simulink model "im1"  (R2018a)
settings: Solver=VariableStepAuto  StartTime=0.0  StopTime=10.0  RelTol=1e-3
values from neighbouring files (symbols this model uses):
  f = 0    [im.m]
  j = 0.011    [im.m]
  k = m/sigma/ls/lr    (= 95.8433439252)    [im.m]
  lambda = rs/sigma/ls+(1-sigma)/sigma/tr    (= 237.19971154)    [im.m]
  lr = 0.1164    [im.m]
  m = 0.1113    [im.m]
  p = 2    [im.m]
  tr = lr/rr    (= 0.111387559809)    [im.m]
settings Model: Creator=Yara  LastModifiedBy=Yara

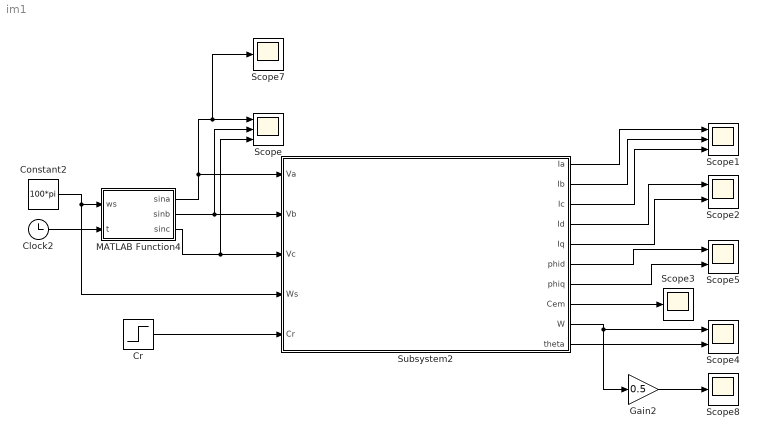
== system im1 ==
  Clock2 : Clock
  Constant2 : Constant  Value=100*pi
  Cr : Step  After=5  SampleTime=0
  Gain2 : Gain  Gain=0.5
  MATLAB Function4 : MATLAB Function  TreatAsAtomicUnit=on
  Scope : Scope  NumInputPorts=3
  Scope1 : Scope  NumInputPorts=3
  Scope2 : Scope  NumInputPorts=2
  Scope3 : Scope
  Scope4 : Scope  NumInputPorts=2
  Scope5 : Scope  NumInputPorts=2
  Scope7 : Scope
  Scope8 : Scope
  Subsystem2 : Subsystem
  wires:
  Subsystem2/5(Iq) -> Scope2/2
  Subsystem2/2(Ib) -> Scope1/2
  Cr/1 -> Subsystem2/5(Cr)
  Subsystem2/8(Cem) -> Scope3/1
  Subsystem2/9(W) -> Scope4/1, Gain2/1
  Subsystem2/7(phiq) -> Scope5/2
  Subsystem2/4(Id) -> Scope2/1
  Subsystem2/6(phid) -> Scope5/1
  Gain2/1 -> Scope8/1
  Subsystem2/1(Ia) -> Scope1/1
  Subsystem2/3(Ic) -> Scope1/3
  Subsystem2/10(theta) -> Scope4/2
  MATLAB Function4/1(sina) -> Subsystem2/1(Va), Scope7/1, Scope/1
  Clock2/1 -> MATLAB Function4/2(t)
  MATLAB Function4/3(sinc) -> Subsystem2/3(Vc), Scope/3
  Constant2/1 -> Subsystem2/4(Ws), MATLAB Function4/1(ws)
  MATLAB Function4/2(sinb) -> Subsystem2/2(Vb), Scope/2

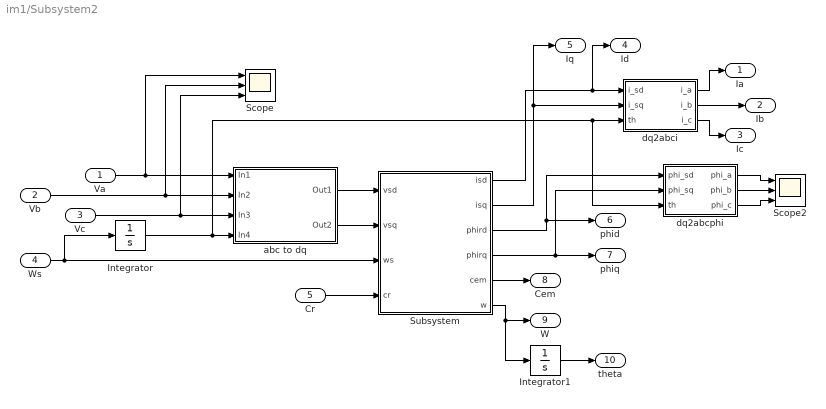
== system im1/Subsystem2 ==
  Va : Inport
  Vb : Inport  Port=2
  Vc : Inport  Port=3
  Ws : Inport  Port=4
  Cr : Inport  Port=5
  Integrator : Integrator
  Integrator1 : Integrator
  Scope : Scope  NumInputPorts=3
  Scope2 : Scope  NumInputPorts=3
  Subsystem : Subsystem
  abc to dq : Subsystem
  dq2abci : MATLAB Function  TreatAsAtomicUnit=on
  dq2abcphi : MATLAB Function  TreatAsAtomicUnit=on
  Ia : Outport
  Ib : Outport  Port=2
  Ic : Outport  Port=3
  Id : Outport  Port=4
  Iq : Outport  Port=5
  phid : Outport  Port=6
  phiq : Outport  Port=7
  Cem : Outport  Port=8
  W : Outport  Port=9
  theta : Outport  Port=10
  wires:
  Vc/1 -> Scope/3, abc to dq/3(In3)
  Subsystem/2(isq) -> Iq/1, dq2abci/2(i_sq)
  dq2abcphi/3(phi_c) -> Scope2/3
  Va/1 -> Scope/1, abc to dq/1(In1)
  dq2abci/2(i_b) -> Ib/1
  Subsystem/6(w) -> Integrator1/1, W/1
  Cr/1 -> Subsystem/4(cr)
  abc to dq/2(Out2) -> Subsystem/2("vsq ")
  Subsystem/4(phirq) -> dq2abcphi/2(phi_sq), phiq/1
  dq2abcphi/2(phi_b) -> Scope2/2
  dq2abcphi/1(phi_a) -> Scope2/1
  dq2abci/1(i_a) -> Ia/1
  dq2abci/3(i_c) -> Ic/1
  Subsystem/1(isd) -> Id/1, dq2abci/1(i_sd)
  Vb/1 -> Scope/2, abc to dq/2(In2)
  Subsystem/3(phird) -> phid/1, dq2abcphi/1(phi_sd)
  abc to dq/1(Out1) -> Subsystem/1(vsd)
  Ws/1 -> Integrator/1, Subsystem/3(ws)
  Integrator1/1 -> theta/1
  Subsystem/5(cem) -> Cem/1
  Integrator/1 -> dq2abcphi/3(th), dq2abci/3(th), abc to dq/4(In4)

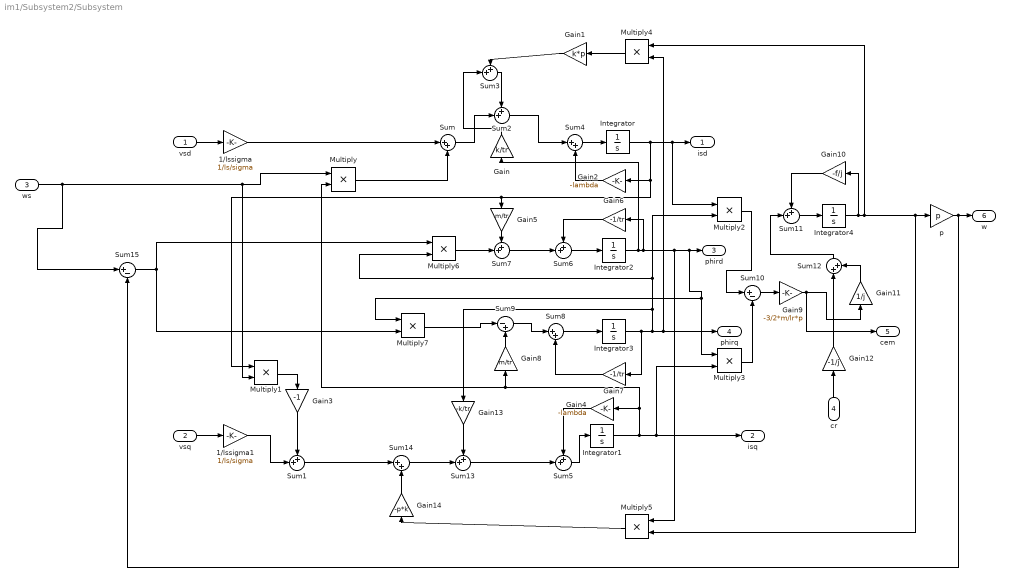
== system im1/Subsystem2/Subsystem ==
  vsd : Inport
  "vsq " : Inport  Port=2
  ws : Inport  Port=3
  cr : Inport  Port=4
  1/lssigma : Gain  Gain=1/ls/sigma
  1/lssigma1 : Gain  Gain=1/ls/sigma
  Gain : Gain  Gain=k/tr
  Gain1 : Gain  Gain=k*p
  Gain10 : Gain  Gain=-f/j
  Gain11 : Gain  Gain=1/j
  Gain12 : Gain  Gain=-1/j
  Gain13 : Gain  Gain=-k/tr
  Gain14 : Gain  Gain=-p*k
  Gain2 : Gain  Gain=-lambda
  Gain3 : Gain  Gain=-1
  Gain4 : Gain  Gain=-lambda
  Gain5 : Gain  Gain=m/tr
  Gain6 : Gain  Gain=-1/tr
  Gain7 : Gain  Gain=-1/tr
  Gain8 : Gain  Gain=m/tr
  Gain9 : Gain  Gain=-3/2*m/lr*p
  Integrator{,1..4} (5 alike) : Integrator
  Multiply{,1..7} (8 alike) : Product
  Sum{,4,8,12,14} (5 alike) : Sum  Inputs=|++
  Sum{1..3,5..7,11,13} (8 alike) : Sum  Inputs=++|
  Sum10 : Sum  Inputs=|+-
  Sum15 : Sum  Inputs=|+-
  Sum9 : Sum  Inputs=|-+
  p : Gain  Gain=p
  isd : Outport
  isq : Outport  Port=2
  phird : Outport  Port=3
  phirq : Outport  Port=4
  cem : Outport  Port=5
  w : Outport  Port=6
  wires:
  vsd/1 -> 1/lssigma/1
  "vsq "/1 -> 1/lssigma1/1
  Sum5/1 -> Integrator1/1
  1/lssigma/1 -> Sum/1
  ws/1 -> Multiply/1, Multiply1/2, Sum15/1
  Multiply/1 -> Sum/2
  1/lssigma1/1 -> Sum1/2
  Sum4/1 -> Integrator/1
  Multiply1/1 -> Gain3/1
  Sum/1 -> Sum2/2
  Gain/1 -> Sum3/2
  Sum3/1 -> Sum2/1
  Gain1/1 -> Sum3/1
  Sum2/1 -> Sum4/1
  Integrator/1 -> Gain2/1, Gain5/1, Multiply1/1, Multiply2/1, isd/1
  Gain2/1 -> Sum4/2
  Gain3/1 -> Sum1/1
  Integrator1/1 -> Gain8/1, Multiply/2, Gain4/1, Multiply3/2, isq/1
  Sum13/1 -> Sum5/2
  Gain4/1 -> Sum5/1
  Sum6/1 -> Integrator2/1
  Gain6/1 -> Sum6/1
  Sum7/1 -> Sum6/2
  Gain5/1 -> Sum7/1
  Sum8/1 -> Integrator3/1
  Gain7/1 -> Sum8/2
  Gain8/1 -> Sum9/2
  Sum9/1 -> Sum8/1
  Multiply2/1 -> Sum10/1
  Multiply3/1 -> Sum10/2
  Sum10/1 -> Gain9/1
  Gain9/1 -> Gain11/1, cem/1
  Sum11/1 -> Integrator4/1
  Gain10/1 -> Sum11/1
  Gain11/1 -> Sum12/2
  Sum12/1 -> Sum11/2
  cr/1 -> Gain12/1
  Gain12/1 -> Sum12/1
  Multiply4/1 -> Gain1/1
  Integrator3/1 -> Gain7/1, Gain13/1, Multiply6/2, Multiply2/2, Multiply4/2, phirq/1
  Gain13/1 -> Sum13/1
  Sum14/1 -> Sum13/2
  Sum1/1 -> Sum14/1
  Gain14/1 -> Sum14/2
  Multiply5/1 -> Gain14/1
  Integrator2/1 -> Multiply5/1, Multiply7/1, Multiply3/1, phird/1, Gain6/1, Gain/1
  Integrator4/1 -> Gain10/1, Multiply4/1, Multiply5/2, p/1
  p/1 -> Sum15/2, w/1
  Sum15/1 -> Multiply7/2, Multiply6/1
  Multiply6/1 -> Sum7/2
  Multiply7/1 -> Sum9/1

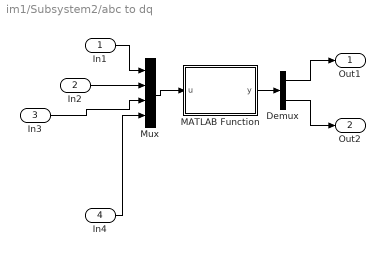
== system im1/Subsystem2/abc to dq ==
  In1 : Inport
  In2 : Inport  Port=2
  In3 : Inport  Port=3
  In4 : Inport  Port=4
  Demux : Demux  Outputs=2
  MATLAB Function : MATLAB Function  TreatAsAtomicUnit=on
  Mux : Mux
  Out1 : Outport
  Out2 : Outport  Port=2
  wires:
  Demux/1 -> Out1/1
  Demux/2 -> Out2/1
  In1/1 -> Mux/1
  In2/1 -> Mux/2
  In3/1 -> Mux/3
  Mux/1 -> MATLAB Function/1(u)
  MATLAB Function/1(y) -> Demux/1
  In4/1 -> Mux/4

== matlab function im1/MATLAB Function4 ==
  data: ws input; sina output; t input; sinb output; sinc output
function [sina,sinb,sinc] = fcn(ws,t)
ph=0.9
A=10.2889;
if(t>=1)
%ws=(5/A+ws/2)*2;
end
V_s=311

sina=V_s*sin(ws*t)
sinb=V_s*sin(ws*t-2*pi/3)
sinc=V_s*sin(ws*t-4*pi/3)
end

== matlab function im1/Subsystem2/dq2abci ==
  data: i_sd input; i_a output; i_sq input; th input; i_b output; i_c output
function [i_a,i_b,i_c] = fcn1(i_sd,i_sq,th)
if isempty(th)
    th=0
end
i_a=sqrt(2/3)*(i_sd*cos(th)-i_sq*sin(th))
i_b=sqrt(2/3)*(i_sd*cos(th-2*pi/3)-i_sq*sin(th-2*pi/3))
i_c=sqrt(2/3)*(i_sd*cos(th-4*pi/3)-i_sq*sin(th-4*pi/3))
end

== matlab function im1/Subsystem2/dq2abcphi ==
  data: phi_sd input; phi_a output; phi_sq input; th input; phi_b output; phi_c output
function [phi_a,phi_b,phi_c] = fcn1(phi_sd,phi_sq,th)

if isempty(th)
    th=0
end


phi_a=sqrt(2/3)*(phi_sd*cos(th)-phi_sq*sin(th))
phi_b=sqrt(2/3)*(phi_sd*cos(th-2*pi/3)-phi_sq*sin(th-2*pi/3))
phi_c=sqrt(2/3)*(phi_sd*cos(th-4*pi/3)-phi_sq*sin(th-4*pi/3))
end

== matlab function im1/Subsystem2/abc to dq/MATLAB Function ==
  data: u input; y output
function y = fcn(u)
th=u(4);
if isempty(th)
    th=0;
end
y=zeros(2,1);
y(1)=sqrt(3/2)*(u(1)*cos(th) +u(2)*cos(th -2*pi/3) +u(3)*cos(th -4*pi/3));
y(2)=sqrt(3/2)*(-u(1)*sin(th) -u(2)*sin(th -2*pi/3) -u(3)*sin(th -4*pi/3));

end
